simulink model "genericActuator"  (R2021b)
settings: Solver=FixedStepDiscrete  StartTime=0.0  StopTime=10.0  FixedStep=sampleTime.hardware  RelTol=1e-3
undefined symbols (not defined in the file or in its folder): sampleTime
libraries: simulink x1
settings Model: Creator=ACH  LastModifiedBy=ACH

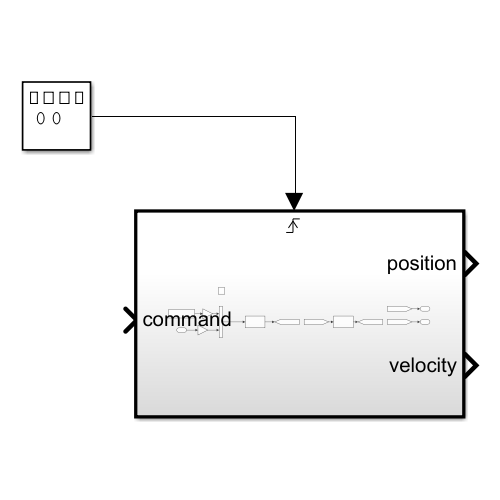
[thumbnail: Simulink's stored preview of the top-level diagram]
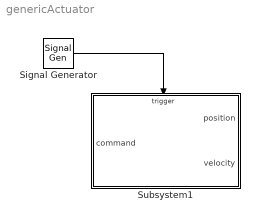
== system genericActuator ==
  Signal Generator : SignalGenerator  WaveForm=square  Frequency=1/sampleTime.hardware  Units=rad/sec
  Subsystem1 : Subsystem
  wires:
  Signal Generator/1 -> Subsystem1/Trigger

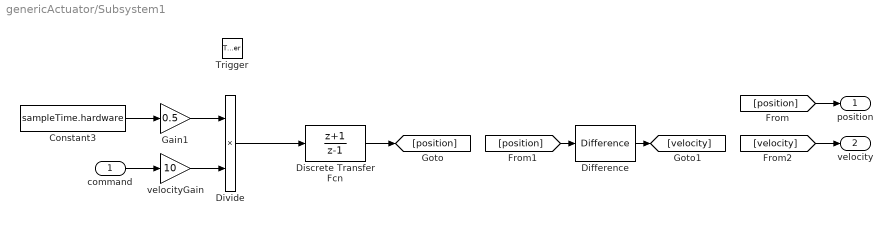
== system genericActuator/Subsystem1 ==
  command : Inport
  Trigger : TriggerPort  VariantControl=(inherit)  PortDimensions=1
  Constant3 : Constant  Value=sampleTime.hardware
  Difference : simulink/Discrete/Difference  ICPrevInput=0.0  OutMin=[]  OutMax=[]  OutDataType=fixdt(1, 16)  OutScaling=2^-10  DoSatur=off
  Discrete Transfer Fcn : DiscreteTransferFcn  Numerator=[1 1]  Denominator=[1 -1]
  Divide : Product  Inputs=**
  Gain1 : Gain  Gain=0.5
  velocityGain : Gain  Gain=10
  position : Outport
  velocity : Outport  Port=2
  wires:
  command/1 -> velocityGain/1
  Gain1/1 -> Divide/1
  Constant3/1 -> Gain1/1
  Divide/1 -> Discrete Transfer Fcn/1
  Discrete Transfer Fcn/1 -> [position]
  [position] -> position/1
  [position] -> Difference/1
  Difference/1 -> [velocity]
  [velocity] -> velocity/1
  velocityGain/1 -> Divide/2
